simulink library "PID_Controller_UL"  (R2019a)
settings: Solver=VariableStepAuto  StartTime=0.0  StopTime=10.0  RelTol=1e-3
undefined symbols (not defined in the file): CTRL
settings Model: Creator=John Jr  LastModifiedBy=John Jr

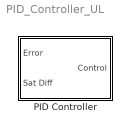
== system PID_Controller_UL ==
  PID Controller : Subsystem  mask{kp=CTRL.Kp, ki=CTRL.Ki, kd=CTRL.Kd, tau=CTRL.tau}
      mask prompts: kp "Proportional gain"; ki "Integral gain"; kd "Derivative gain"; tau "Filter time constant"
      mask DialogControl DescGroupVar Prompt: Filtered PID Controller
      mask DialogControl DescTextVar Prompt: This block models a filtered PID controller with anti-windup.
      mask DialogControl Control2 Prompt: Controller Parameters:
      mask Display:
      | patch([0 1 1 0], [0 0 1 1],[.8 1 1])
      | 
      | port_label('input',1,'\fontname{Cambria Math}Error','texmode','on')
      | port_label('input',2,'\fontname{Cambria Math}Sat Diff','texmode','on')
      | 
      | port_label('output',1,'\fontname{Cambria Math}Control','texmode','on')

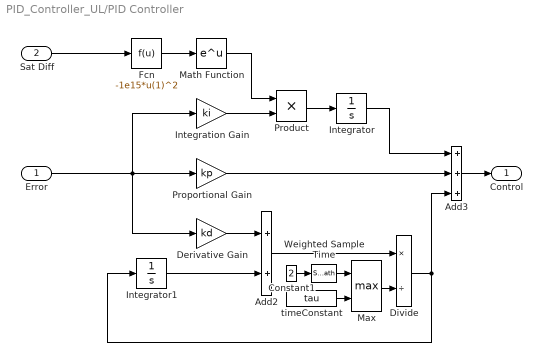
== system PID_Controller_UL/PID Controller ==
  Error : Inport
  Sat Diff : Inport  Port=2
  Add2 : Sum
  Add3 : Sum  Inputs=+++
  Constant1 : Constant  Value=2
  Derivative Gain : Gain  Gain=kd
  Divide : Product  Inputs=*/
  Fcn : Fcn  Expr=-1e15*u(1)^2
  Integration Gain : Gain  Gain=ki
  Integrator : Integrator
  Integrator1 : Integrator
  Math Function : Math  SaturateOnIntegerOverflow=on
  Max : MinMax  Function=max  Inputs=2
  Product : Product
  Proportional Gain : Gain  Gain=kp
  Weighted Sample Time : SampleTimeMath  TsampMathOp=Ts Only  weightValue=1
  timeConstant : Constant  Value=tau
  Control : Outport
  wires:
  Add3/1 -> Control/1
  Fcn/1 -> Math Function/1
  Error/1 -> Derivative Gain/1, Proportional Gain/1, Integration Gain/1
  Sat Diff/1 -> Fcn/1
  Math Function/1 -> Product/1
  Proportional Gain/1 -> Add3/2
  Product/1 -> Integrator/1
  Integrator/1 -> Add3/1
  Integration Gain/1 -> Product/2
  timeConstant/1 -> Max/2
  Max/1 -> Divide/2
  Constant1/1 -> Weighted Sample Time/1
  Integrator1/1 -> Add2/2
  Add2/1 -> Divide/1
  Weighted Sample Time/1 -> Max/1
  Derivative Gain/1 -> Add2/1
  Divide/1 -> Integrator1/1, Add3/3
